simulink model "SpeedToPulse"  (R2017b)
settings: Solver=FixedStepDiscrete  StartTime=0.0  StopTime=10000  FixedStep=1  RelTol=1e-3
libraries: simulink x1, hdlsllib x1
settings Model: Creator=chandler.ga  LastModifiedBy=Gavin
settings CodeAppCC: StateflowObjectComments=on

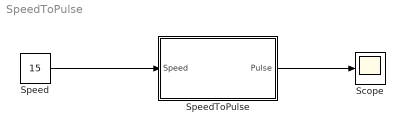
== system SpeedToPulse ==
  Scope : Scope
  Speed : Constant  Value=15  OutDataTypeStr=uint8
  SpeedToPulse : Subsystem
  wires:
  Speed/1 -> SpeedToPulse/1(Speed)
  SpeedToPulse/1(Pulse) -> Scope/1

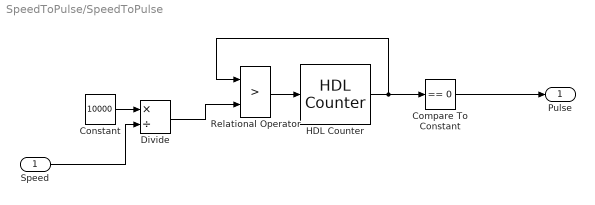
== system SpeedToPulse/SpeedToPulse ==
  Speed : Inport  OutDataTypeStr=uint8
  Compare To Constant : simulink/Logic and Bit Operations/Compare To Constant  relop===  const=0  OutDataTypeStr=boolean
  Constant : Constant  Value=10000
  Divide : Product  Inputs=*/  SaturateOnIntegerOverflow=on  RndMeth=Zero
  HDL Counter : hdlsllib/Sources/HDL Counter  CountType=Count limited  CountInit=0  CountStep=1  CountMax=10000  CountFromType=Initial value  CountFrom=0  CountResetPort=on  CountLoadPort=off  CountEnbPort=off  CountDirPort=off  CountDataType=Unsigned  CountWordLen=18  CountFracLen=0  CountSampTime=1
      settings: SourceProductBaseCode=HD
  Relational Operator : RelationalOperator  Operator=>  OutDataTypeStr=boolean  RndMeth=Nearest
  Pulse : Outport
  wires:
  Constant/1 -> Divide/1
  HDL Counter/1 -> Relational Operator/1, Compare To Constant/1
  Divide/1 -> Relational Operator/2
  Speed/1 -> Divide/2
  Compare To Constant/1 -> Pulse/1
  Relational Operator/1 -> HDL Counter/1
